simulink model "main"  (R2022a)
settings: Solver=FixedStepDiscrete  StartTime=0.0  StopTime=Inf  FixedStep=(50e-6)-(sim_en*4.995e-5)  RelTol=1e-3  EnableMultiTasking=on
model workspace (MAT data in the model file):
  Param : Simulink.Parameter (value not decoded)
  ac_ok : Simulink.Signal (value not decoded)
  ac_ok_120 : Simulink.Signal (value not decoded)
  bulk_voltage : Simulink.Signal (value not decoded)
  burstduty_integ_max : Simulink.Signal (value not decoded)
  burstduty_integ_min : Simulink.Signal (value not decoded)
  burstduty_ki : Simulink.Signal (value not decoded)
  burstduty_kp : Simulink.Signal (value not decoded)
  calib_ok : Simulink.Signal (value not decoded)
  can_addr1 : Simulink.Signal (value not decoded)
  can_addr2 : Simulink.Signal (value not decoded)
  can_addr3 : Simulink.Signal (value not decoded)
  can_addr4 : Simulink.Signal (value not decoded)
  can_data_rx : Simulink.Signal (value not decoded)
  can_data_tx : Simulink.Signal (value not decoded)
  can_timeout_120 : Simulink.Signal (value not decoded)
  chksum_scircv : Simulink.Signal (value not decoded)
  clllc_en_120 : Simulink.Signal (value not decoded)
  clllc_fault_120 : Simulink.Signal (value not decoded)
  clllc_ok_120 : Simulink.Signal (value not decoded)
  cmpss1h : Simulink.Signal (value not decoded)
  cmpss1l : Simulink.Signal (value not decoded)
  cmpss2h : Simulink.Signal (value not decoded)
  cmpss2l : Simulink.Signal (value not decoded)
  cmpss3h : Simulink.Signal (value not decoded)
  cmpss3l : Simulink.Signal (value not decoded)
  cmpss4h : Simulink.Signal (value not decoded)
  cmpss4l : Simulink.Signal (value not decoded)
  cmpss5h : Simulink.Signal (value not decoded)
  cmpss5l : Simulink.Signal (value not decoded)
  cmpss6h : Simulink.Signal (value not decoded)
  cmpss6l : Simulink.Signal (value not decoded)
  cmpss7h : Simulink.Signal (value not decoded)
  cmpss7l : Simulink.Signal (value not decoded)
  cmpss8h : Simulink.Signal (value not decoded)
  cmpss8l : Simulink.Signal (value not decoded)
  cnt_idle : Simulink.Signal (value not decoded)
  cnt_orps : Simulink.Signal (value not decoded)
  cnt_scircv : Simulink.Signal (value not decoded)
  cnt_scixmt : Simulink.Signal (value not decoded)
  cnt_scixmt_func : Simulink.Signal (value not decoded)
  cnt_temp_mux : Simulink.Signal (value not decoded)
  cnt_vdroop : Simulink.Signal (value not decoded)
  config_ok : Simulink.Signal (value not decoded)
  control_en : Simulink.Signal (value not decoded)
  cp_ready_120 : Simulink.Signal (value not decoded)
  d2d_en : Simulink.Signal (value not decoded)
  dchg_off : Simulink.Signal (value not decoded)
  debug_dacb : Simulink.Signal (value not decoded)
  debug_dacc : Simulink.Signal (value not decoded)
  debug_msg1 : Simulink.Signal (value not decoded)
  debug_msg2 : Simulink.Signal (value not decoded)
  debug_msg3 : Simulink.Signal (value not decoded)
  debug_msg4 : Simulink.Signal (value not decoded)
  debug_msg5 : Simulink.Signal (value not decoded)
  debug_msg6 : Simulink.Signal (value not decoded)
  dir_v2g : Simulink.Signal (value not decoded)
  eoss_llc1 : Simulink.Signal (value not decoded)
  eoss_llc2 : Simulink.Signal (value not decoded)
  eoss_orps : Simulink.Signal (value not decoded)
  fault_ocp : Simulink.Signal (value not decoded)
  fault_otp : Simulink.Signal (value not decoded)
  fault_ovp : Simulink.Signal (value not decoded)
  fut_en : Simulink.Signal (value not decoded)
  fwd_en_120 : Simulink.Signal (value not decoded)
  gain_llc1_sec_idc : Simulink.Signal (value not decoded)
  gain_llc1_temp_sr : Simulink.Signal (value not decoded)
  gain_llc2_sec_idc : Simulink.Signal (value not decoded)
  gain_vbat : Simulink.Signal (value not decoded)
  gain_vbulk : Simulink.Signal (value not decoded)
  gain_vout : Simulink.Signal (value not decoded)
  input_current_phasea : Simulink.Signal (value not decoded)
  input_current_phaseb : Simulink.Signal (value not decoded)
  input_current_phasec : Simulink.Signal (value not decoded)
  input_freq : Simulink.Signal (value not decoded)
  input_power : Simulink.Signal (value not decoded)
  input_voltage_phasea : Simulink.Signal (value not decoded)
  input_voltage_phaseb : Simulink.Signal (value not decoded)
  input_voltage_phasec : Simulink.Signal (value not decoded)
  ishare_arbiter : Simulink.Signal (value not decoded)
  ishare_thresh : Simulink.Signal (value not decoded)
  led_g : Simulink.Signal (value not decoded)
  led_r : Simulink.Signal (value not decoded)
  led_y : Simulink.Signal (value not decoded)
  llc1_burst_integ : Simulink.Signal (value not decoded)
  llc1_burstduty_buffer : Simulink.Signal (value not decoded)
  llc1_pfm_error : Simulink.Signal (value not decoded)
  llc1_pfm_integ : Simulink.Signal (value not decoded)
  llc1_pfm_prop : Simulink.Signal (value not decoded)
  llc1_pri_idc : Simulink.Signal (value not decoded)
  llc1_ps_buffer : Simulink.Signal (value not decoded)
  llc1_pspwm_error : Simulink.Signal (value not decoded)
  llc1_pspwm_integ : Simulink.Signal (value not decoded)
  llc1_pspwm_prop : Simulink.Signal (value not decoded)
  llc1_sec_idc : Simulink.Signal (value not decoded)
  llc1_temp_sr : Simulink.Signal (value not decoded)
  llc1_ts_tbctr_buffer : Simulink.Signal (value not decoded)
  llc2_burst_integ : Simulink.Signal (value not decoded)
  llc2_burstduty_buffer : Simulink.Signal (value not decoded)
  llc2_en : Simulink.Signal (value not decoded)
  llc2_en_buffer : Simulink.Signal (value not decoded)
  llc2_pfm_error : Simulink.Signal (value not decoded)
  llc2_pfm_integ : Simulink.Signal (value not decoded)
  llc2_pfm_prop : Simulink.Signal (value not decoded)
  llc2_pri_idc : Simulink.Signal (value not decoded)
  llc2_ps_buffer : Simulink.Signal (value not decoded)
  llc2_pspwm_error : Simulink.Signal (value not decoded)
  llc2_pspwm_integ : Simulink.Signal (value not decoded)
  llc2_pspwm_prop : Simulink.Signal (value not decoded)
  llc2_sec_idc : Simulink.Signal (value not decoded)
  llc2_temp_sr : Simulink.Signal (value not decoded)
  llc2_ts_tbctr_buffer : Simulink.Signal (value not decoded)
  loop_adcint : Simulink.Signal (value not decoded)
  loop_control : Simulink.Signal (value not decoded)
  loop_idle : Simulink.Signal (value not decoded)
  mid_bulk_voltage : Simulink.Signal (value not decoded)
  mode_120 : Simulink.Signal (value not decoded)
  mode_cc_cv : Simulink.Signal (value not decoded)
  myParam : mpt.Parameter (value not decoded)
  obc_ok_120 : Simulink.Signal (value not decoded)
  offset_llc1_sec_idc : Simulink.Signal (value not decoded)
  offset_llc1_temp_sr : Simulink.Signal (value not decoded)
  offset_llc2_sec_idc : Simulink.Signal (value not decoded)
  offset_vbat : Simulink.Signal (value not decoded)
  offset_vbulk : Simulink.Signal (value not decoded)
  offset_vout : Simulink.Signal (value not decoded)
  openloop_en : Simulink.Signal (value not decoded)
  openloop_fault_en : Simulink.Signal (value not decoded)
  ot_fault_120 : Simulink.Signal (value not decoded)
  pfc_en : Simulink.Signal (value not decoded)
  pfc_en_120 : Simulink.Signal (value not decoded)
  pfc_fw_revision : Simulink.Signal (value not decoded)
  pfc_fw_revision_bootloader : Simulink.Signal (value not decoded)
  pfc_fw_revision_debug : Simulink.Signal (value not decoded)
  pfc_ok : Simulink.Signal (value not decoded)
  pfc_ok_120 : Simulink.Signal (value not decoded)
  pfm_a0 : Simulink.Signal (value not decoded)
  pfm_a1 : Simulink.Signal (value not decoded)
  pfm_integ_max : Simulink.Signal (value not decoded)
  pfm_integ_min : Simulink.Signal (value not decoded)
  pfm_ki : Simulink.Signal (value not decoded)
  pfm_kp : Simulink.Signal (value not decoded)
  pri_fut_en : Simulink.Signal (value not decoded)
  pri_fut_en_buffer : Simulink.Signal (value not decoded)
  pri_halfbridge_en : Simulink.Signal (value not decoded)
  pri_halfbridge_en_buffer : Simulink.Signal (value not decoded)
  pspwm_integ_max : Simulink.Signal (value not decoded)
  pspwm_integ_min : Simulink.Signal (value not decoded)
  pspwm_ki : Simulink.Signal (value not decoded)
  pspwm_kp : Simulink.Signal (value not decoded)
  ref_idclink_max : Simulink.Signal (value not decoded)
  ref_iout : Simulink.Signal (value not decoded)
  ref_iout_calib : Simulink.Signal (value not decoded)
  ref_iout_llc1 : Simulink.Signal (value not decoded)
  ref_iout_llc1_calib : Simulink.Signal (value not decoded)
  ref_iout_llc2 : Simulink.Signal (value not decoded)
  ref_iout_llc2_calib : Simulink.Signal (value not decoded)
  ref_pout : Simulink.Signal (value not decoded)
  ref_ss_llc1 : Simulink.Signal (value not decoded)
  ref_ss_llc2 : Simulink.Signal (value not decoded)
  ref_ss_orps : Simulink.Signal (value not decoded)
  ref_vbat : Simulink.Signal (value not decoded)
  ref_vbat_calib : Simulink.Signal (value not decoded)
  ref_vbulk : Simulink.Signal (value not decoded)
  ref_vbulk_calib : Simulink.Signal (value not decoded)
  ref_vbulk_llc1_calib : Simulink.Signal (value not decoded)
  ref_vbulk_llc2_calib : Simulink.Signal (value not decoded)
  ref_vout : Simulink.Signal (value not decoded)
  ref_vout_calib : Simulink.Signal (value not decoded)
  relay_en : Simulink.Signal (value not decoded)
  reset_flag : Simulink.Signal (value not decoded)
  rev_en_120 : Simulink.Signal (value not decoded)
  runtime_control : Simulink.Signal (value not decoded)
  runtime_idle : Simulink.Signal (value not decoded)
  scircv_buffer : Simulink.Signal (value not decoded)
  scircv_buffer_tmp : Simulink.Signal (value not decoded)
  scircv_buffer_tmp_idx0 : Simulink.Signal (value not decoded)
  scircv_chksum : Simulink.Signal (value not decoded)
  scircv_chksum_ok : Simulink.Signal (value not decoded)
  scircv_parse_ok : Simulink.Signal (value not decoded)
  scixmt_buffer : Simulink.Signal (value not decoded)
  scixmt_chksum : Simulink.Signal (value not decoded)
  scixmt_func : Simulink.Signal (value not decoded)
  scixmt_word0_lsb : Simulink.Signal (value not decoded)
  scixmt_word0_msb : Simulink.Signal (value not decoded)
  scixmt_word1_lsb : Simulink.Signal (value not decoded)
  scixmt_word1_msb : Simulink.Signal (value not decoded)
  scixmt_word2_lsb : Simulink.Signal (value not decoded)
  scixmt_word2_msb : Simulink.Signal (value not decoded)
  scixmt_wr : Simulink.Signal (value not decoded)
  ss_step : Simulink.Signal (value not decoded)
  state_calib : Simulink.Signal (value not decoded)
  state_control : Simulink.Signal (value not decoded)
  state_hkeep : Simulink.Signal (value not decoded)
  status_cmpss : Simulink.Signal (value not decoded)
  status_control : Simulink.Signal (value not decoded)
  status_digin : Simulink.Signal (value not decoded)
  status_digout : Simulink.Signal (value not decoded)
  status_fault : Simulink.Signal (value not decoded)
  status_input : Simulink.Signal (value not decoded)
  status_pfc : Simulink.Signal (value not decoded)
  temp_inlet : Simulink.Signal (value not decoded)
  temp_llc1_fet_hs : Simulink.Signal (value not decoded)
  temp_llc2_fet_hs : Simulink.Signal (value not decoded)
  temp_mux : Simulink.Signal (value not decoded)
  temp_mux_s0 : Simulink.Signal (value not decoded)
  temp_mux_s1 : Simulink.Signal (value not decoded)
  temp_mux_s2 : Simulink.Signal (value not decoded)
  temp_outlet : Simulink.Signal (value not decoded)
  temp_pfc_fet_hsa : Simulink.Signal (value not decoded)
  temp_pfc_fet_hsb : Simulink.Signal (value not decoded)
  temp_pfc_fet_hsc : Simulink.Signal (value not decoded)
  temp_pfc_fet_lsa : Simulink.Signal (value not decoded)
  temp_pfc_fet_lsb : Simulink.Signal (value not decoded)
  temp_pfc_fet_lsc : Simulink.Signal (value not decoded)
  test_mode : Simulink.Signal (value not decoded)
  tfcv_cc : Simulink.Signal (value not decoded)
  tfcv_cc_llc2 : Simulink.Signal (value not decoded)
  tfcv_cv : Simulink.Signal (value not decoded)
  tfcv_sr_en : Simulink.Signal (value not decoded)
  tfv_assert_llc1_pri_idc : Simulink.Signal (value not decoded)
  tfv_assert_llc1_sec_idc : Simulink.Signal (value not decoded)
  tfv_assert_llc1_temp_sr : Simulink.Signal (value not decoded)
  tfv_assert_llc2_pri_idc : Simulink.Signal (value not decoded)
  tfv_assert_llc2_sec_idc : Simulink.Signal (value not decoded)
  tfv_assert_llc2_temp_sr : Simulink.Signal (value not decoded)
  tfv_assert_temp_outlet : Simulink.Signal (value not decoded)
  tfv_assert_vaux_uv : Simulink.Signal (value not decoded)
  tfv_assert_vbat : Simulink.Signal (value not decoded)
  tfv_assert_vbulk : Simulink.Signal (value not decoded)
  tfv_assert_vout : Simulink.Signal (value not decoded)
  tfv_cnt_tz : Simulink.Signal (value not decoded)
  tfv_deassert_llc1_pri_idc : Simulink.Signal (value not decoded)
  tfv_deassert_llc1_sec_idc : Simulink.Signal (value not decoded)
  tfv_deassert_llc1_temp_sr : Simulink.Signal (value not decoded)
  tfv_deassert_llc2_pri_idc : Simulink.Signal (value not decoded)
  tfv_deassert_llc2_sec_idc : Simulink.Signal (value not decoded)
  tfv_deassert_llc2_temp_sr : Simulink.Signal (value not decoded)
  tfv_deassert_temp_outlet : Simulink.Signal (value not decoded)
  tfv_deassert_vaux_uv : Simulink.Signal (value not decoded)
  tfv_deassert_vbat : Simulink.Signal (value not decoded)
  tfv_deassert_vbulk : Simulink.Signal (value not decoded)
  tfv_deassert_vout : Simulink.Signal (value not decoded)
  tfv_llc1_pri_idc : Simulink.Signal (value not decoded)
  tfv_llc1_sec_idc : Simulink.Signal (value not decoded)
  tfv_llc1_temp_sr : Simulink.Signal (value not decoded)
  tfv_llc2_pri_idc : Simulink.Signal (value not decoded)
  tfv_llc2_sec_idc : Simulink.Signal (value not decoded)
  tfv_llc2_temp_sr : Simulink.Signal (value not decoded)
  tfv_temp_outlet : Simulink.Signal (value not decoded)
  tfv_vaux_uv : Simulink.Signal (value not decoded)
  tfv_vbat : Simulink.Signal (value not decoded)
  tfv_vbulk : Simulink.Signal (value not decoded)
  tfv_vout : Simulink.Signal (value not decoded)
  timer_1ms : Simulink.Signal (value not decoded)
  tz : Simulink.Signal (value not decoded)
  valve_en : Simulink.Signal (value not decoded)
  vaux : Simulink.Signal (value not decoded)
  vbat : Simulink.Signal (value not decoded)
  vbulk : Simulink.Signal (value not decoded)
  vout : Simulink.Signal (value not decoded)
undefined symbols (not defined in the file or in its folder): CAN_O_INT, CANA_BASE, Down, GPTRIP1SEL, GPTRIP2SEL, TZ1, TZ2, Up
libraries: hdlsllib x159, simulink x100, c2837xDlib x24, c2807xlib x16, c280xlib x13, c2802xlib x12, canmsglib x8, idelinklib_common x2, c2000lib x1, c281xlib x1
(part 15 of 15)

== stateflow chart main/Control_State_Machine/Control_Loop/control ==
  note: Reset / Init
  note: Openloop
  state tzClear [function]
  state disClb [function]
  note: System State
      |
      | 0 - Sleep
      | 1 - Standby
      | 2 - Forward Start
      | 3 - Forward Run
      | 4 - Reverse Start
      | 5 - Reverse Run
      | 6 - Fault Reset
      | 7 - Fault Latch
      | 8 - Test Mode
  note: Config
  state INIT
    du:
    resetControlParam();
    disClb();
    disPwm();
    tzClear();
    PFC_EN = false;
    OBC_OK = false;
    state_control = 0;  // Init System State to Sleep
  state disPwm [function]
  state configSr(dir_v2g) [function] [commented out]
  state resetControlParam [function]
  state disableSR [function]
  state SLEEP
    en:
    du:
    state_control = 0;  //System in Sleep
  state enableSR [function]
  note: Closed Loop
  state TEST_MODE
    note: PWM_ON
    note: PWM OFF
    (default) -> (junction 4260)
    (junction 4260) -> (junction 4261) [order 2] : {state_control = 9;}
    (junction 4260) -> (junction 4261) [order 1] : [u8ModeCmd == 0xA4]
        | {state_control = 8;}
    (junction 4261) -> (junction 4262) [order 1] : [u8OpenLoopEn1==0]
    (junction 4261) -> (junction 4661) [order 2]
    (junction 4262) -> (junction 4264) : {
        | disPwm();
        | loop_enx = 0;
        | }
    (junction 4661) -> (junction 4263) [order 2]
    (junction 4661) -> (junction 4658) [order 1] : [loop_enx == 0]
        | {
        | loop_enx = 1;
        | //init Open Loop Paramters
        | llc1_burstduty = 100; //100% Burst
        | llc1_ps = 0; //0% Phase Shift
        | llc1_ts_tbctr = 333; //300Khz
        | //init Past Values
        | ol_llc1burstdty_past = llc1_burstduty;
        | ol_llc1ps_past = llc1_ps;
        | ol_llc1tstbctr_past = llc1_ts_tbctr;
        | }
    (junction 4263) -> (junction 4668) [order 2]
    (junction 4263) -> (junction 4665) [order 1] : [f32BurstDuty1 != ol_llc1burstdty_past]
    (junction 4665) -> (junction 4668) [order 3] : {ol_llc1burstdty_past = 0;}
    (junction 4665) -> (junction 4668) [order 1] : [f32BurstDuty1 > ol_llc1burstdty_past]
        | {
        |    ol_llc1burstdty_past += 0.25;
        | }
    (junction 4665) -> (junction 4668) [order 2] : [f32BurstDuty1 < ol_llc1burstdty_past  &&  ol_llc1burstdty_past > 0.25]
        | {
        |    ol_llc1burstdty_past -= 0.25;
        | }
    (junction 4668) -> (junction 4674)
    (junction 4674) -> (junction 4677) [order 2]
    (junction 4674) -> (junction 4675) [order 1] : [f32PhaseShift1 != ol_llc1ps_past]
    (junction 4675) -> (junction 4677) [order 3] : {ol_llc1ps_past = 0;}
    (junction 4675) -> (junction 4677) [order 1] : [f32PhaseShift1 > ol_llc1ps_past]
        | {
        |    ol_llc1ps_past += 0.25;
        | }
    (junction 4675) -> (junction 4677) [order 2] : [f32PhaseShift1 < ol_llc1ps_past &&  ol_llc1ps_past > 0.25]
        | {
        |    ol_llc1ps_past -= 0.25;
        | }
    (junction 4677) -> (junction 4689)
    (junction 4689) -> (junction 4686) [order 2]
    (junction 4689) -> (junction 4685) [order 1] : [f32FreqPeriod1 != ol_llc1tstbctr_past]
    (junction 4685) -> (junction 4686) [order 3] : {ol_llc1tstbctr_past = 333;}
    (junction 4685) -> (junction 4686) [order 1] : [f32FreqPeriod1 > ol_llc1tstbctr_past]
        | {
        |    ol_llc1tstbctr_past += 0.25;
        | }
    (junction 4685) -> (junction 4686) [order 2] : [f32FreqPeriod1 < ol_llc1tstbctr_past &&  ol_llc1tstbctr_past > 333.25]
        | {
        |    ol_llc1tstbctr_past -= 0.25;
        | }
    (junction 4686) -> (junction 4692) : {
        | llc1_burstduty = ol_llc1burstdty_past;
        | llc1_ps = ol_llc1ps_past;
        | llc1_ts_tbctr = ol_llc1tstbctr_past;
        | }
    (junction 4658) -> (junction 4265)
    (junction 4264) -> (junction 4265)
    (junction 4692) -> (junction 4265) [order 2] : {disableSR();}
    (junction 4692) -> (junction 4265) [order 1] : [llc1_ps == 0 && llc1_burstduty == 100 && llc1_ts_tbctr > 333]
        | {
        | enableSR();
        | }
  note: Note: Exit only for Trip Zone Fault
  note: Forward
  note: Reverse
  note: Init Control Parameters
  state STANDBY
    en:
    PFC_EN = false;
    OBC_OK = false;
    CLLLC_OK = false;
    disPwm();
    tzClear();
    disClb();
    resetControlParam();
    sSecFault = 0x0000;
    precharge_count=0;
    modeswitch_count=0;
    ss_stepcount=0;
    loop_enx = 0;
    du:
    state_control = 1; //System in Standby
  state initG2vCvPfm [function]
  state initV2gCvPfm [function]
  state initV2gCvPspwm [function]
  state initG2vCvPspwm [function]
  state initV2gCvBurst [function]
  state initG2vCvBurst [function]
  state initG2vCcPfm [function]
  state REVERSE_START
    en:
    state_control = 4; //System in Reverse Start State
    du:
  state FORWARD_START
    en:
    PFC_EN = true;
    state_control = 2; //System in Forward Start State
    du:
  state initG2vCcPspwm [function]
  state initG2vCcBurst [function]
  note: Find Operating Mode (CC or CV) / Limits
  state tfv_status = tfcvCv(input, assert_lim, assert_vld, deassert_lim, deassert_vld) [function]
  state tfv_status = tfcvCc(input, assert_lim, assert_vld, deassert_lim, deassert_vld) [function]
  state REVERSE_RUN
    (default) -> (junction 4720)
    (junction 4720) -> (junction 4712) [order 1] : [(precharge_count <4000)]
        | {precharge_count = precharge_count +1;
        | state_control = 5;}
    (junction 4712) -> (junction 4714) [order 1] : [vbulk>=ref_vbulk_calib]{
        | llc1_burstduty = 0;
        | llc1_burstduty_integ = 0;
        | }
    (junction 4712) -> (junction 4714) [order 2] : [llc1_burstduty <100]
        | {llc1_burstduty = llc1_burstduty+0.4;
        | //0.025 changed to 0.25 to change 0.4
        | llc1_burstduty_integ = llc1_burstduty;
        | }
    (junction 4712) -> (junction 4714) [order 3] : {llc1_burstduty = 100;
        | llc1_burstduty_integ = 100;
        | }
    (junction 4720) -> (junction 4723) [order 2] : {state_control = 5;}
    (junction 4723) -> (junction 4729) [order 1] : [loop_enx == 0]
        | {
        | initV2gCvBurst();
        | initV2gCvPspwm();
        | initV2gCvPfm();
        | loop_enx = 1;
        | ref = vbulk;
        | }
    (junction 4723) -> (junction 4729) [order 2]
    (junction 4729) -> (junction 4714) : {
        | llcControlLoopwithSS(ref_vbulk_calib,vbulk,15);
        | mode_cc_cv=1;
        | OBC_OK = true;
        | //200V/S SS Step rate => 15
        | }
    (junction 4714) -> (junction 4724)
  state FORWARD_RUN
    (default) -> (junction 4280)
    (junction 4280) -> (junction 4454) [order 1] : [(precharge_count <4000)]
        | {precharge_count = precharge_count +1;
        | state_control = 3;}
    (junction 4454) -> (junction 4286) [order 3] : {llc1_burstduty = 100;
        | llc1_burstduty_integ = 100;
        | }
    (junction 4454) -> (junction 4286) [order 2] : [llc1_burstduty <100]
        | {llc1_burstduty = llc1_burstduty+0.4; //0.025 changed to 0.25 to change 0.4
        | llc1_burstduty_integ = llc1_burstduty;
        | }
    (junction 4454) -> (junction 4286) [order 1] : [vbat>=ref_vbat_calib]{
        | llc1_burstduty = 0;
        | llc1_burstduty_integ = 0;
        | }
    (junction 4280) -> (junction 4547) [order 2] : {tfcv_cv = tfcvCv(vbat,ref_vbat_calib, uint16(10), ref_vout_calib - 80, uint16(10));
        | tfcv_cc = tfcvCc(llc1_sec_idc, ref_iout_llc1_calib,  uint16(5), ref_iout_llc1_calib*0.9, uint16(5));
        | state_control = 3;}
    (junction 4547) -> (junction 4629) [order 1] : [mode_cc_cv== 0]
    (junction 4547) -> (junction 4634) [order 2]
    (junction 4634) -> (junction 4636) [order 1] : [loop_enx == 0]
        | {
        | initG2vCvBurst();
        | initG2vCvPspwm();
        | initG2vCvPfm();
        | loop_enx = 1;
        | ref = vbat;
        | }
    (junction 4629) -> (junction 4632) [order 1] : [loop_enx == 0]
        | {
        | initG2vCcBurst();
        | initG2vCcPspwm();
        | initG2vCcPfm();
        | loop_enx = 1;
        | ref = llc1_sec_idc;
        | }
    (junction 4629) -> (junction 4632) [order 2]
    (junction 4634) -> (junction 4636) [order 2]
    (junction 4636) -> (junction 4558) : {
        | llcControlLoopwithSS(ref_vbat_calib,vbat,15);
        | //200V/S SS Step rate => 15
        | }
    (junction 4632) -> (junction 4557) : {
        | llcControlLoopwithSS(ref_iout_llc1_calib,llc1_sec_idc,39);
        | //20A/S SS Step rate = 39
        | }
    (junction 4557) -> (junction 4554) [order 2]
    (junction 4558) -> (junction 4554) [order 2]
    (junction 4558) -> (junction 4554) [order 1] : [!tfcv_cv && tfcv_cc ]
        | {
        | mode_cc_cv = 0;
        | loop_enx = 0;
        | }
    (junction 4557) -> (junction 4554) [order 1] : [tfcv_cv]
        | {
        | mode_cc_cv = 1;
        | loop_enx = 0;
        | }
    (junction 4554) -> (junction 4286) : {OBC_OK = true;}
    (junction 4286) -> (junction 4288)
  state ref_pout = configPowerLimitG2v(ref_vbat, ref_iout) [function] [commented out]
  note: Control Loop
  state llcControlLoopwithSS(ref_calib,fb,ss_stepdelay) [function]
    note: SOFT START
    note: BURST
    note: PSPWM
    note: PFM
    (default) -> (junction 4641)
    (junction 4641) -> (junction 4642) [order 1] : [!eoss_llc1 || ref != ref_calib]
    (junction 4641) -> (junction 4381) [order 2]
    (junction 4642) -> (junction 4381) [order 1] : [ss_stepcount < ss_stepdelay]
        | {
        | ss_stepcount+=1;
        | }
    (junction 4642) -> (junction 4382) [order 2] : {
        | ss_stepcount = 0;
        | diff = ref_calib - ref;
        | }
    (junction 4382) -> (junction 4654) [order 3]
    (junction 4382) -> (junction 4386) [order 1] : [diff > 1]
    (junction 4382) -> (junction 4650) [order 2] : [diff < -1]
    (junction 4654) -> (junction 4648) : {
        | ref = ref_calib;
        | eoss_llc1 = 1
        | }
    (junction 4386) -> (junction 4648) : {
        | ref = ref + 1;
        | eoss_llc1 = 0;
        | }
    (junction 4650) -> (junction 4648) : {
        | ref = ref-1;
        | eoss_llc1 = 0;
        | }
    (junction 4648) -> (junction 4381)
    (junction 4381) -> (junction 4568)
    (junction 4572) -> (junction 4576) [order 2] : {modeswitch_count = 0;}
    (junction 4568) -> (junction 4572) [order 1] : [mode == 0]
        | {[llc1_burstduty, llc1_burstduty_integ] = burstLlc1(ref,fb,llc1_burstduty_integ);}
    (junction 4568) -> (junction 4584) [order 2] : [mode == 1]
        | {disableSR();
        | [llc1_ps, llc1_ps_integ] = pspwmLlc1(ref, fb,llc1_ps_integ);
        | }
    (junction 4568) -> (junction 4609) [order 4]
    (junction 4568) -> (junction 4605) [order 3] : [mode == 2]
        | {enableSR();
        |  llc1_ts_tbctr = pfmLlc1(ref, fb, llc1_pfm_integral);
        | llc1_pfm_integral = llc1_ts_tbctr;
        | }
    (junction 4572) -> (junction 4574) [order 1] : [llc1_burstduty>=100 && fb < ref]
    (junction 4574) -> (junction 4576) [order 2] : {modeswitch_count++;}
    (junction 4576) -> (junction 4602)
    (junction 4574) -> (junction 4576) [order 1] : [modeswitch_count >= 5]
        | {mode = 1; //Switch to PSPWM
        | modeswitch_count = 0;
        | llc1_ps_integ = 36;
        | }
    (junction 4602) -> (junction 4600)
    (junction 4584) -> (junction 4600) [order 3] : {modeswitch_count = 0;}
    (junction 4584) -> (junction 4586) [order 1] : [llc1_ps<=pspwm_integ_min && fb<ref]
    (junction 4584) -> (junction 4591) [order 2] : [llc1_ps>=pspwm_integ_max && fb>ref]
    (junction 4600) -> (junction 4596)
    (junction 4591) -> (junction 4593) [order 2] : {modeswitch_count++;}
    (junction 4586) -> (junction 4588) [order 2] : {modeswitch_count++;}
    (junction 4591) -> (junction 4593) [order 1] : [modeswitch_count >= 5]
        | {mode = 0; //Switch to Burst
        | modeswitch_count = 0;
        | llc1_burstduty_integ = 100;
        | }
    (junction 4586) -> (junction 4588) [order 1] : [modeswitch_count >= 5]
        | {mode = 2; //Switch to PFM
        | modeswitch_count = 0;
        | llc1_pfm_integral = 333;
        | }
    (junction 4593) -> (junction 4596)
    (junction 4588) -> (junction 4596)
    (junction 4596) -> (junction 4609)
    (junction 4605) -> (junction 4618) [order 2] : {modeswitch_count = 0;}
    (junction 4605) -> (junction 4616) [order 1] : [llc1_ts_tbctr<=pfm_integ_min && fb>ref]
    (junction 4616) -> (junction 4618) [order 2] : {modeswitch_count++;}
    (junction 4616) -> (junction 4618) [order 1] : [modeswitch_count >=5]
        | {mode = 1; //Switch to PSPWM
        | modeswitch_count = 0;
        | llc1_ps_integ = 36;
        | }
    (junction 4618) -> (junction 4609)
    (junction 4609) -> (junction 4607)
  state llc1_ts_tbctr = pfmLlc1(ref,input,pfm_integ_in) [function]
  note: Note:
      | Exit from Reset Mode only when Fault Flags gets Resets
  state [llc1_ps,pspwm_integ_out] = pspwmLlc1(ref,input,pspwm_integ_in) [function]
  state FAULT_RESET
    en:
    state_control = 6;
  state [llc1_burstduty,burstduty_integ_out] = burstLlc1(ref,input,burstduty_integ_in) [function]
  state FAULT_LATCH
    en:
    state_control = 7;
  (default) -> INIT
  INIT -> SLEEP : [state_control == 0]
  STANDBY -> TEST_MODE [order 3] : [u8ModeCmd == 0xA4 || u8ModeCmd == 0xA5]
  STANDBY -> SLEEP [order 1] : [u8ModeCmd == 0xA0]
  SLEEP -> STANDBY : [u8ModeCmd == 0xA1]
  TEST_MODE -> FAULT_LATCH [order 2] : [sSecFault & 0x0080 != 0]
      | {disPwm();}
  TEST_MODE -> STANDBY [order 1] : [u8ModeCmd == 0xA0 || u8ModeCmd == 0xA1]
  TEST_MODE -> TEST_MODE [order 3]
  FAULT_LATCH -> STANDBY : [u8ModeCmd == 0xA1|| u8ModeCmd == 0xA0]
  STANDBY -> REVERSE_START [order 4] : [u8ModeCmd == 0xA3 && sSecFault == 0]
  STANDBY -> FORWARD_START [order 2] : [AC_OK == true && CP_READY == true && u8ModeCmd == 0xA2 && sSecFault == 0 ]
  REVERSE_START -> STANDBY [order 2] : [u8ModeCmd == 0xA1|| u8ModeCmd == 0xA0]
  (junction 4311) -> STANDBY
  FORWARD_START -> STANDBY [order 1] : [AC_OK == false || CP_READY == false || u8ModeCmd == 0xA1|| u8ModeCmd == 0xA0]
  REVERSE_START -> REVERSE_RUN [order 1] : [CLLLC_EN == true]
  FORWARD_START -> FORWARD_RUN [order 2] : [PFC_OK == true]
  REVERSE_RUN -> REVERSE_RUN [order 4]
  FORWARD_RUN -> FORWARD_RUN [order 4]
  REVERSE_RUN -> (junction 4311) [order 2] : [CLLLC_EN == false || u8ModeCmd == 0xA1 || u8ModeCmd == 0xA0 ]
      | { CLLLC_OK  = false; OBC_OK = false;  disPwm(); state_control = 1;}
  FORWARD_RUN -> (junction 4311) [order 1] : [CP_READY == false || PFC_OK == false || u8ModeCmd == 0xA1 || u8ModeCmd == 0xA0 ]
      |                                      { PFC_EN = false; OBC_OK = false; disPwm();  state_control = 1;}
  FAULT_RESET -> (junction 4311) : [sSecFault == 0]
  FORWARD_RUN -> FAULT_LATCH [order 3] : [sSecFault & 0x0081 != 0]
      | {disPwm(); PFC_EN = false; OBC_OK = false;}
  FORWARD_RUN -> FAULT_RESET [order 2] : [sSecFault & 0x307E != 0]
      | {disPwm(); PFC_EN = false; OBC_OK = false;}
  REVERSE_RUN -> FAULT_LATCH [order 3] : [sSecFault & 0x0081 != 0]
      | {disPwm(); CLLLC_OK  = false; OBC_OK = false;}
  REVERSE_RUN -> FAULT_RESET [order 1] : [sSecFault & 0x3F70 != 0]
      | {disPwm(); CLLLC_OK  = false; OBC_OK = false;}
  data: dir_v2g function_input double size=1; tfv_status function_output boolean; input function_input uint16 size=1; assert_lim function_input uint16 size=1; assert_vld function_input uint16 size=1; deassert_lim function_input uint16 size=1; deassert_vld function_input uint16 size=1; tfv_status function_output boolean; input function_input uint16 size=1; assert_lim function_input uint16 size=1; assert_vld function_input uint16 size=1; deassert_lim function_input uint16 size=1; deassert_vld function_input uint16 size=1; ref_vbat function_input double size=1; ref_iout function_input double size=1; ref_pout function_output double size=1; ref_calib function_input double; fb function_input double; diff local double; ss_stepdelay function_input uint16; ref function_input; input function_input; llc1_ts_tbctr function_output; pfm_integ_in function_input; ref function_input; input function_input; llc1_ps function_output; pspwm_integ_in function_input; pspwm_integ_out function_output; ref function_input; input function_input; llc1_burstduty function_output; burstduty_integ_in function_input single; burstduty_integ_out function_output single; llc1_sec_idc data_store_memory; dir_v2g data_store_memory; status_digin data_store_memory; openloop_en data_store_memory; pfc_ok data_store_memory; pfc_en data_store_memory; state_control data_store_memory; tfv_vbulk data_store_memory; tfcv_cc data_store_memory; eoss_llc1 data_store_memory; ref_iout data_store_memory; ref_vbat data_store_memory; vbat data_store_memory; vbulk data_store_memory; llc1_ts_tbctr data_store_memory; ref_ss_llc1 local uint16; llc1_ps data_store_memory; ref_vbulk data_store_memory; control_en data_store_memory; vout data_store_memory; ac_ok data_store_memory; ref_iout_calib data_store_memory; ref_vbat_calib data_store_memory; ref_vbulk_calib data_store_memory; status_control data_store_memory; sSecFault data_store_memory; status_digout data_store_memory; status_cmpss data_store_memory; calib_ok data_store_memory; pspwm_kp data_store_memory; pspwm_ki data_store_memory; pfm_kp data_store_memory; pfm_ki data_store_memory; pfm_integ_max data_store_memory; pfm_integ_min data_store_memory; pspwm_integ_max data_store_memory; pspwm_integ_min data_store_memory; ss_step data_store_memory; burstduty_integ_max data_store_memory; llc1_burstduty data_store_memory; config_ok data_store_memory; pri_halfbridge_en data_store_memory; llc1_pfm_integ data_store_memory; llc1_burst_integ data_store_memory; llc1_pspwm_integ data_store_memory; relay_en data_store_memory; ref_iout_llc1_calib data_store_memory; pri_halfbridge_en_buffer data_store_memory; llc1_pri_idc data_store_memory; ref_vbulk_llc1_calib data_store_memory; openloop_fault_en data_store_memory; ref_pout data_store_memory; tfv_vbat data_store_memory; ref_idclink_max data_store_memory; cnt_vdroop local uint16 =0; llc1_vbulk local uint16; runtime_control data_store_memory; fut_en data_store_memory; state_hkeep data_store_memory; gain_vout data_store_memory; gain_vbat data_store_memory; ref_ss_orps data_store_memory; eoss_orps data_store_memory; cnt_orps data_store_memory; gain_vbulk data_store_memory; valve_en data_store_memory; mcu_en local boolean =1; reset_flag data_store_memory; mode data_store_memory; eoss local double; loop_en local double; fbk local single; loop_enx data_store_memory; ref data_store_memory; ref_c local single; ref_vout_calib data_store_memory; ref_vout data_store_memory; u16Debug1 data_store_memory; u8OpenLoopEn1 data_store_memory; tfv_llc1_sec_idc data_store_memory; tfv_vout data_store_memory; tz_oc data_store_memory; tfv_llc1_pri_idc data_store_memory; tz_ov data_store_memory; tfcv_cv data_store_memory; test_mode data_store_memory; u8ModeCmd data_store_memory; mode_cc_cv data_store_memory; CP_READY input; AC_OK input; PFC_OK input; PFC_EN output double; OBC_OK output double; CLLLC_OK output double; CLLLC_EN input; precharge_count data_store_memory; modeswitch_count data_store_memory; llc1_burstduty_integ data_store_memory; ss_stepcount data_store_memory; ol_llc1burstdty_past local single =0; ol_llc1tstbctr_past local single =333; ol_llc1ps_past local single =0; f32PhaseShift1 data_store_memory; f32FreqPeriod1 data_store_memory; f32BurstDuty1 data_store_memory; llc1_ps_integ data_store_memory; llc1_pfm_integral data_store_memory

== stateflow chart main/Task_Manager/idle/idle_task/comm_npc/comm_npc ==
  state COMM_NPC
    //du:
    //readScircvBuffer1();
    note: SCIXMT
    state calcScixmtChksum [function]
    state packScixmt(scixmt_chksum) [function]
    state sendScixmt(scixmt_buffer, cnt_scixmt) [function]
    state INIT
      en:
      /*scixmt*/
      cnt_scixmt = 0;
      scixmt_chksum = 0;
      /*scircv*/
      scircv_parse_ok = false;
      scircv_chksum_ok = false;
      scircv_chksum = 0;
    state PARSE_SCIRCV
      en:
      scircv_parse_ok = parseScircv(scircv_buffer_tmp);
    note: SCIRCV
    state scircv_parse_ok = parseScircv(scircv_buffer_tmp) [function]
    state calcScircvChksum(scircv_buffer) [function]
    state VERIFY_CHKSUM_SCIRCV
      en:
      calcScircvChksum(scircv_buffer);
      scircv_chksum_ok = verifyScircvChksum(scircv_chksum);
    state scircv_chksum_ok = verifyScircvChksum(scircv_chksum) [function]
    state PACK_SCIXMT
      en:
      //parseScixmtWr(scixmt_wr);
      calcScixmtChksum();
      packScixmt(scixmt_chksum);
    state extractScircv(scircv_buffer) [function]
    state scixmt_func = incrFunc(cnt_scixmt_func) [function]
    state EXTRACT_SCIRCV
      en:
      extractScircv(scircv_buffer);
      scixmt_func = incrFunc(cnt_scixmt_func);
    state readScircvBuffer [function] [commented out]
    state SEND_SCIXMT
      en:
      sendScixmt(scixmt_buffer, cnt_scixmt);
    state readScircvBuffer1 [function] [commented out]
    EXTRACT_SCIRCV -> INIT
    VERIFY_CHKSUM_SCIRCV -> INIT [order 2]
    (default) -> INIT
    PARSE_SCIRCV -> INIT [order 2]
    SEND_SCIXMT -> PARSE_SCIRCV [order 2]
    PARSE_SCIRCV -> VERIFY_CHKSUM_SCIRCV [order 1] : [scircv_parse_ok]
    INIT -> PACK_SCIXMT
    VERIFY_CHKSUM_SCIRCV -> EXTRACT_SCIRCV [order 1] : [scircv_chksum_ok]
    PACK_SCIXMT -> SEND_SCIXMT
    SEND_SCIXMT -> SEND_SCIXMT [order 1] : [cnt_scixmt < 11]
        | {cnt_scixmt = cnt_scixmt + 1;}
  data: scixmt_chksum function_input; scixmt_buffer function_input uint8; cnt_scixmt function_input uint8; scircv_parse_ok function_output; scircv_buffer_tmp function_input; scircv_buffer function_input; scircv_chksum_ok function_output boolean; scircv_chksum function_input; scircv_buffer function_input; cnt_scixmt_func function_input; scixmt_func function_output; cnt_scircv data_store_memory; scixmt_buffer data_store_memory; cnt_scixmt data_store_memory; scircv_buffer_tmp data_store_memory; control_en data_store_memory; scircv_buffer data_store_memory; scixmt_word0_lsb data_store_memory; scixmt_chksum data_store_memory; scixmt_func data_store_memory; scixmt_wr data_store_memory; scircv_chksum_ok data_store_memory; scircv_parse_ok data_store_memory; scircv_chksum data_store_memory; scixmt_word0_msb data_store_memory; scixmt_word1_lsb data_store_memory; scixmt_word1_msb data_store_memory; scixmt_word2_msb data_store_memory; scixmt_word2_lsb data_store_memory; cnt_scixmt_func data_store_memory

== stateflow chart main/Task_Manager/idle/idle_task/hkeep/tfv/hkeep ==
  state HKEEP
    du:
    //tfv_vout = tfvVout(vout, tfv_assert_vout, uint16(100), tfv_deassert_vout, uint16(100));
    tfv_vbat = tfvVbat(vout, tfv_assert_vbat, uint16(100), tfv_deassert_vbat, uint16(100));
    tfv_vbulk = tfvVbulk(vbulk, tfv_assert_vbulk, uint16(100), tfv_deassert_vbulk, uint16(100));
    //tfv_vaux_uv = tfvVauxUvp(vaux, tfv_assert_vaux_uv, uint16(100), tfv_deassert_vaux_uv, uint16(100));
    //tfv_temp_outlet = tfvTempOutlet(temp_outlet, tfv_assert_temp_outlet, uint16(2000), tfv_deassert_temp_outlet, uint16(2000));
    note: General Protections
    state INIT
      en:
      state_hkeep = 0;
    state tfv_status = tfvVout(input, assert_lim, assert_vld, deassert_lim, deassert_vld) [function] [commented out]
    state tfv_status = tfvVbat(input, assert_lim, assert_vld, deassert_lim, deassert_vld) [function]
    state tfv_status = tfvVbulk(input, assert_lim, assert_vld, deassert_lim, deassert_vld) [function]
    state tfv_status = tfvTempOutlet(input,assert_lim,assert_vld,deassert_lim,deassert_vld) [function] [commented out]
    state G2V
      en:
      state_hkeep = 1;
      du:
      tfv_llc1_sec_idc = tfvLlc1SecIdc(llc1_sec_idc, tfv_assert_llc1_sec_idc, uint16(20), tfv_deassert_llc1_sec_idc, uint16(20));
      //tfv_llc1_temp_sr = tfvLlc1TempSr(llc1_temp_sr, tfv_assert_llc1_temp_sr, uint16(2000), tfv_deassert_llc1_temp_sr, uint16(2000));
    state V2G [commented out]
      en:
      state_hkeep = 2;
      du:
      tfv_llc1_pri_idc = tfvLlc1PriIdc(llc1_pri_idc, tfv_assert_llc1_pri_idc, uint16(20), tfv_deassert_llc1_pri_idc, uint16(20));
    state tfv_status = tfvVauxUvp(input,assert_lim,assert_vld,deassert_lim,deassert_vld) [function] [commented out]
    note: G2V Protections
    state tfv_status = tfvLlc1SecIdc(input,assert_lim,assert_vld,deassert_lim,deassert_vld) [function]
    state tfv_status = tfvLlc1TempSr(input,assert_lim,assert_vld,deassert_lim,deassert_vld) [function] [commented out]
    note: V2G Protections
    state tfv_status = tfvLlc1PriIdc(input,assert_lim,assert_vld,deassert_lim,deassert_vld) [function] [commented out]
    (default) -> INIT
    INIT -> V2G [commented out]
    INIT -> G2V : [!dir_v2g]
    V2G -> G2V [commented out] : [!dir_v2g && !status_fault]
    G2V -> V2G [commented out] : [dir_v2g && !status_fault]
  data: tfv_status function_output double size=1; input function_input double size=1; assert_lim function_input double size=1; assert_vld function_input double size=1; deassert_lim function_input double size=1; deassert_vld function_input double size=1; tfv_status function_output boolean; input function_input uint16 size=1; assert_lim function_input uint16 size=1; assert_vld function_input uint16 size=1; deassert_lim function_input uint16 size=1; deassert_vld function_input uint16 size=1; tfv_status function_output boolean; input function_input uint16 size=1; assert_lim function_input uint16 size=1; assert_vld function_input uint16 size=1; deassert_lim function_input uint16 size=1; deassert_vld function_input uint16 size=1; tfv_status function_output double size=1; input function_input double size=1; assert_lim function_input double size=1; assert_vld function_input double size=1; deassert_lim function_input double size=1; deassert_vld function_input double size=1; tfv_status function_output double size=1; input function_input double size=1; assert_lim function_input double size=1; assert_vld function_input double size=1; deassert_lim function_input double size=1; deassert_vld function_input double size=1; tfv_status function_output boolean; input function_input uint16 size=1; assert_lim function_input uint16 size=1; assert_vld function_input uint16 size=1; deassert_lim function_input uint16 size=1; deassert_vld function_input uint16 size=1; tfv_status function_output double size=1; input function_input double size=1; assert_lim function_input double size=1; assert_vld function_input double size=1; deassert_lim function_input double size=1; deassert_vld function_input double size=1; tfv_status function_output double size=1; input function_input double size=1; assert_lim function_input double size=1; assert_vld function_input double size=1; deassert_lim function_input double size=1; deassert_vld function_input double size=1; tfv_vout local double; tfv_llc1_sec_idc data_store_memory; llc1_sec_idc data_store_memory; tfv_vout data_store_memory; tfv_vbat data_store_memory; vout data_store_memory; vbat data_store_memory; ref_vbat data_store_memory; tfv_assert_vbat data_store_memory; tfv_assert_llc1_sec_idc data_store_memory; tfv_deassert_llc1_sec_idc data_store_memory; tfv_deassert_vbat data_store_memory; llc1_temp_sr data_store_memory; tfv_assert_llc1_temp_sr data_store_memory; tfv_deassert_llc1_temp_sr data_store_memory; tfv_llc1_temp_sr data_store_memory; tfv_assert_vout data_store_memory; tfv_deassert_vout data_store_memory; tfv_vbulk data_store_memory; dir_v2g data_store_memory; tfv_assert_vbulk data_store_memory; tfv_deassert_vbulk data_store_memory; vbulk data_store_memory; tfcv_cv data_store_memory; status_fault data_store_memory; state_hkeep data_store_memory; llc2_temp_sr data_store_memory; llc2_sec_idc data_store_memory; tfv_deassert_llc2_temp_sr data_store_memory; tfv_deassert_llc2_sec_idc data_store_memory; tfv_assert_llc2_temp_sr data_store_memory; tfv_assert_llc2_sec_idc data_store_memory; tfv_llc2_sec_idc data_store_memory; tfv_llc2_temp_sr data_store_memory; status_control data_store_memory; llc1_pri_idc data_store_memory; llc2_pri_idc data_store_memory; tfv_assert_llc1_pri_idc data_store_memory; tfv_assert_llc2_pri_idc data_store_memory; tfv_deassert_llc1_pri_idc data_store_memory; tfv_deassert_llc2_pri_idc data_store_memory; tfv_llc1_pri_idc data_store_memory; tfv_llc2_pri_idc data_store_memory; tfv_assert_temp_outlet data_store_memory; tfv_deassert_temp_outlet data_store_memory; tfv_temp_outlet data_store_memory; tfv_vaux_uv data_store_memory; tfv_deassert_vaux_uv data_store_memory; tfv_assert_vaux_uv data_store_memory; vaux data_store_memory; temp_outlet data_store_memory

== stateflow chart main/interrupt_adcd/burst_control/burst ==
  state BURST_DIS
    en:
    disPwm();
  state disPwm [function]
  state disPulse [function]
  state enPulse [function]
  state BURST_EN
    state PWM_DIS
      en:
      cnt_pwm_dis+=1;
      disPulse();
    state PWM_EN
      en:
      cnt_pwm_en+=1;
      enPulse();
    (default) -> (junction 1681)
    PWM_EN -> (junction 1681) [order 1] : [cnt_pwm_en>=(burst_pulses_buffer)]
    (junction 1681) -> PWM_EN [order 2] : {cnt_pwm_dis=0;
        | cnt_pwm_en=0;
        | burst_pulses_buffer=burst_pulses;}
    (junction 1681) -> PWM_DIS [order 1] : [burst_pulses_buffer!=16]
        | {cnt_pwm_dis=0;
        | cnt_pwm_en=0;
        | burst_pulses_buffer=burst_pulses;}
    PWM_DIS -> (junction 1681) [order 1] : [cnt_pwm_dis>=16]
    PWM_DIS -> PWM_EN [order 2] : [cnt_pwm_dis>=(16-burst_pulses_buffer)]
    PWM_DIS -> PWM_DIS [order 3]
    PWM_EN -> PWM_EN [order 2]
  (default) -> BURST_DIS
  BURST_DIS -> BURST_EN : [(state_control ==3) || (state_control ==5) || (((state_control ==8) || (state_control ==9)) && (u8OpenLoopEn1 == 1)) ]
  BURST_EN -> BURST_DIS : [(state_control ==1) || (state_control ==2) || (state_control ==6) || (state_control ==7) || (((state_control ==8) || (state_control ==9)) && (u8OpenLoopEn1 == 0))]
  data: control_en data_store_memory; cnt_pwm_en local uint16 =0; cnt_pwm_dis local uint16 =0; burst_pulses input int8; burst_pulses_buffer local int8; pri_halfbridge_en data_store_memory; config_ok data_store_memory; state_control data_store_memory; status_fault data_store_memory; u8OpenLoopEn1 data_store_memory; sSecFault data_store_memory; u8ModeCmd data_store_memory

== stateflow chart main/50e-6 ==
  state INIT
    en:
    sim_control;
  (default) -> INIT
  INIT -> INIT
  events: sim_control output FUNCTION_CALL_EVENT
